simulink model "GRAL_diferentziazko_EK_eta_simulazioa"  (R2015b)
settings: Solver=FixedStepAuto  StartTime=0.0  StopTime=20  FixedStep=Auto  RelTol=1e-3
values from neighbouring files (symbols this model uses):
  g = -9.8    [GRAL_diferentziazko_ekuzaioa.m]
  L = 46    [GRAL_diferentziazko_ekuzaioa.m]
  R = 5.65    [GRAL_diferentziazko_ekuzaioa.m]
  T = 0.0529    [GRAL_diferentziazko_ekuzaioa.m]
undefined symbols (not defined in the file or in its folder): deno, nume
libraries: simulink x1
settings Model: Creator=Pavilion  LastModifiedBy=Pavilion

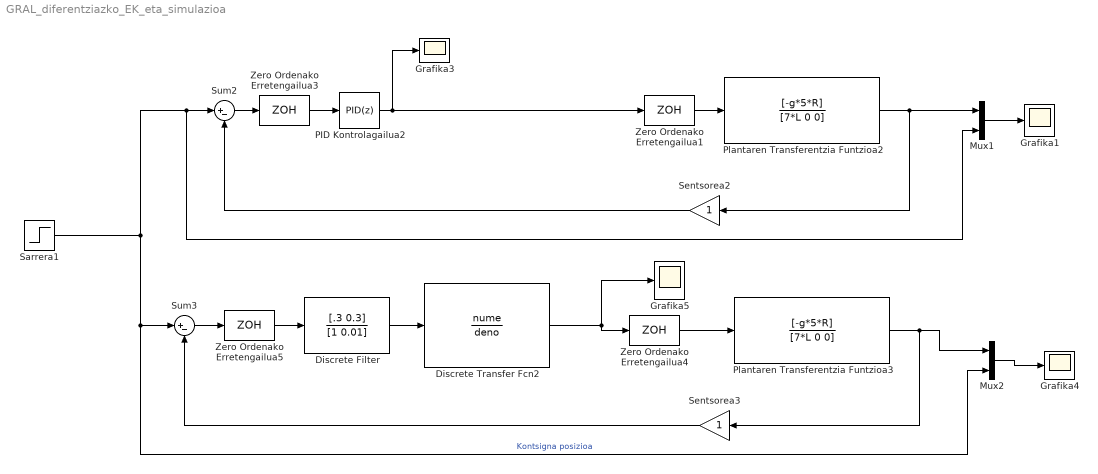
== system GRAL_diferentziazko_EK_eta_simulazioa ==
  Discrete Transfer Fcn2 : DiscreteTransferFcn  Numerator=nume  Denominator=deno
  Discrete Filter : DiscreteFilter  Numerator=[.3 0.3]  Denominator=[1 0.01]  InputProcessing=Columns as channels (frame based)  FilterStructure=Direct form II transposed  a0EqualsOne=on
  Grafika{1,3..5} (4 alike) : Scope
  Mux1 : Mux  Inputs=2
  Mux2 : Mux  Inputs=2
  PID Kontrolagailua2 : simulink/Continuous/PID Controller  Controller=PID  TimeDomain=Discrete-time  SampleTime=-1  IntegratorMethod=Trapezoidal  FilterMethod=Forward Euler  Form=Parallel  UseFilter=off  ControllerParametersSource=internal  P=9.69983864863877  I=0.583196187001297  D=40.332426679988  N=34.7347128437765  InitialConditionSource=internal  InitialConditionForIntegrator=0  InitialConditionForFilter=0  ExternalReset=none  LimitOutput=off  UpperSaturationLimit=90  LowerSaturationLimit=-90  LinearizeAsGain=on  AntiWindupMode=none  Kb=1  TrackingMode=off  Kt=1  PParamMin=[]  PParamMax=[]  IParamMin=[]  IParamMax=[]  DParamMin=[]  DParamMax=[]  NParamMin=[]  NParamMax=[]  KbParamMin=[]  KbParamMax=[]  KtParamMin=[]  KtParamMax=[]  POutMin=[]  POutMax=[]  IOutMin=[]  IOutMax=[]  DOutMin=[]  DOutMax=[]  NOutMin=[]  NOutMax=[]  KbOutMin=[]  KbOutMax=[]  KtOutMin=[]  KtOutMax=[]  IntegratorOutMin=[]  IntegratorOutMax=[]  FilterOutMin=[]  FilterOutMax=[]  SumOutMin=[]  SumOutMax=[]  SumI1OutMin=[]  SumI1OutMax=[]  SumI2OutMin=[]  SumI2OutMax=[]  SumI3OutMin=[]  SumI3OutMax=[]  SumDOutMin=[]  SumDOutMax=[]  SaturationOutMin=[]  SaturationOutMax=[]  IntegratorContinuousStateAttributes=''  IntegratorStateMustResolveToSignalObject=off  IntegratorRTWStateStorageClass=Auto  FilterContinuousStateAttributes=''  FilterStateMustResolveToSignalObject=off  FilterRTWStateStorageClass=Auto  DifferentiatorICPrevScaledInput=0  DifferentiatorOutMin=[]  DifferentiatorOutMax=[]
  Plantaren Transferentzia Funtzioa2 : TransferFcn  Numerator=[-g*5*R]  Denominator=[7*L 0 0]
  Plantaren Transferentzia Funtzioa3 : TransferFcn  Numerator=[-g*5*R]  Denominator=[7*L 0 0]
  Sarrera1 : Step  After=20  SampleTime=0
  Sentsorea2 : Gain
  Sentsorea3 : Gain
  Sum2 : Sum  Inputs=|+-
  Sum3 : Sum  Inputs=|+-
  Zero Ordenako Erretengailua{1,3..5} (4 alike) : ZeroOrderHold  SampleTime=T
  wires:
  Mux1/1 -> Grafika1/1
  Plantaren Transferentzia Funtzioa2/1 -> Sentsorea2/1, Mux1/1
  Zero Ordenako Erretengailua1/1 -> Plantaren Transferentzia Funtzioa2/1
  Sentsorea2/1 -> Sum2/2
  Sum2/1 -> Zero Ordenako Erretengailua3/1
  Zero Ordenako Erretengailua3/1 -> PID Kontrolagailua2/1
  Mux2/1 -> Grafika4/1
  Plantaren Transferentzia Funtzioa3/1 -> Sentsorea3/1, Mux2/1
  Zero Ordenako Erretengailua4/1 -> Plantaren Transferentzia Funtzioa3/1
  Sentsorea3/1 -> Sum3/2
  Sum3/1 -> Zero Ordenako Erretengailua5/1
  Zero Ordenako Erretengailua5/1 -> Discrete Filter/1
  Discrete Filter/1 -> Discrete Transfer Fcn2/1
  Discrete Transfer Fcn2/1 -> Grafika5/1, Zero Ordenako Erretengailua4/1
  Sarrera1/1 -> Mux1/2, Sum2/1, Sum3/1, Mux2/2  "Kontsigna posizioa"
  PID Kontrolagailua2/1 -> Grafika3/1, Zero Ordenako Erretengailua1/1
